simulink model "dpgonio"  (R2019a)
settings: Solver=FixedStepAuto  StartTime=0.0  StopTime=25  RelTol=1e-3  EnableMultiTasking=on
undefined symbols (not defined in the file): Pull, Ts, up
libraries: speedgoatlib_IO183 x5, slrtlib x3, simulink x2
settings Model: Creator=vnalam  LastModifiedBy=vnalam
settings SolverCC: ConcurrentTasks=on  AutoInsertRateTranBlk=on
settings DataIOCC: SaveFormat=StructureWithTime
settings OptimizationCC: BlockReduction=off  OptimizeBlockIOStorage=off  BufferReuse=off  GlobalBufferReuse=off  ExpressionFolding=off  LocalBlockOutputs=off  OptimizeDataStoreBuffers=off  BusAssignmentInplaceUpdate=off
settings HardwareCC: ProdBitPerPointer=32  ProdBitPerSizeT=32  ProdBitPerPtrDiffT=32  ProdLargestAtomicFloat=None  ProdWordSize=32  ProdLongLongMode=on  ProdHWDeviceType=Generic->32-bit x86 compatible
settings RTWCC: SystemTargetFile=slrt.tlc  TemplateMakefile=slrt_default_tmf  Description=Simulink Real-Time  CodeExecutionProfiling=on  RTWCompilerOptimization=on
settings SimulinkRealTimeCC: SupportVariableSizeSignals=on  PreserveStateflowLocalDataDimensions=off  RL32LogTETModifier=off  xPCisDownloadable=off  xPCConcurrentTasks=on

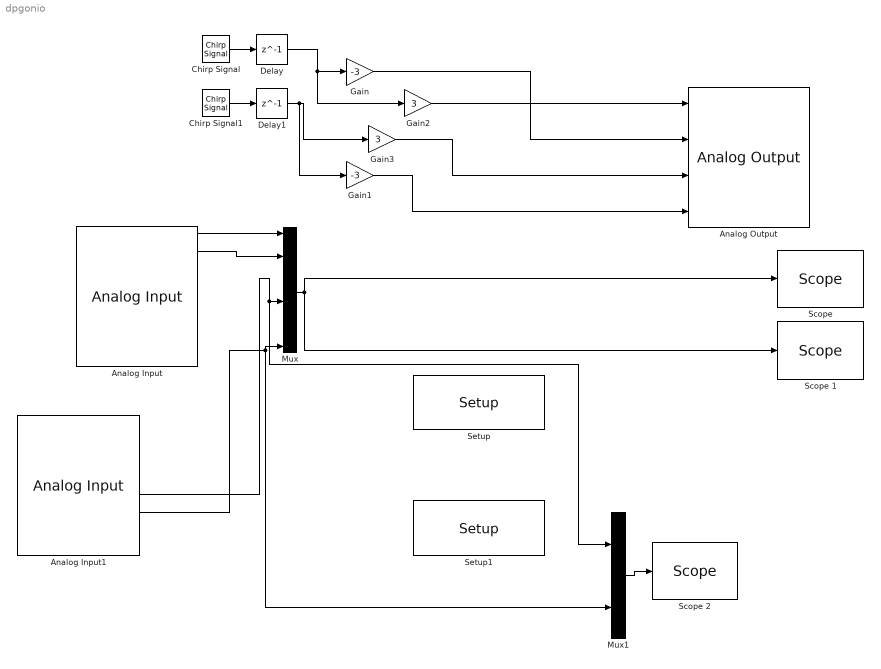
== system dpgonio ==
  Analog Input : speedgoatlib_IO183/Analog Input  Priority=0  parModuleId=1  parSampTime=Ts  parPciSlot=-1  parAdChannelLow=1  parAdChannelHigh=8
      settings: SourceProductName=Simulink Real-Time: Speedgoat Library
  Analog Input1 : speedgoatlib_IO183/Analog Input  Priority=0  parModuleId=2  parSampTime=Ts  parPciSlot=-1  parAdChannelLow=1  parAdChannelHigh=8
      settings: SourceProductName=Simulink Real-Time: Speedgoat Library
  Analog Output : speedgoatlib_IO183/Analog Output  parModuleId=1  parSampTime=-1  parDaSimult=on  parPciSlot=-1  parDaChannels=[1 2 3 4]  parDaInit=[0 0 0 0]  parDaReset=[0 0 0 0]
      settings: SourceProductName=Simulink Real-Time: Speedgoat Library
  Chirp Signal : simulink/Sources/Chirp Signal  f1=0.6  T=25  f2=0.8
  Chirp Signal1 : simulink/Sources/Chirp Signal  f1=0.6  T=25  f2=0.8
  Delay : Delay  DelayLength=1  InitialCondition=0  SampleTime=Ts
  Delay1 : Delay  DelayLength=1  InitialCondition=0  SampleTime=Ts
  Gain : Gain  Gain=-3
  Gain1 : Gain  Gain=-3
  Gain2 : Gain  Gain=3
  Gain3 : Gain  Gain=3
  Mux : Mux  Inputs=6
  Mux1 : Mux  Inputs=2
  "Scope " : slrtlib/Displays and Logging/Scope   scopeno=1  scopetype=Target  autostart=on  viewmode=Graphical sliding  formatstr='%15.6f'  grid=on  ylimits=[0,0]  nosamples=80000  noprepostsamples=0  interleave=1  triggermode=FreeRun  triggersignal=1  trigsignalfromport=off  triggerlevel=0.0  triggerslope=Either  triggerscope=1  triggersample=0  filename=data.dat  mode=Lazy  writesize=512  autorestart=off  dynamicfilemode=off  maxwritefilesize=512*1024^2
  Scope 1 : slrtlib/Displays and Logging/Scope   scopeno=2  scopetype=File  autostart=on  viewmode=Graphical redraw  formatstr='%15.6f'  grid=on  ylimits=[0,0]  nosamples=60000  noprepostsamples=0  interleave=1  triggermode=FreeRun  triggersignal=1  trigsignalfromport=off  triggerlevel=0.0  triggerslope=Either  triggerscope=1  triggersample=0  filename=DPfoot.dat  mode=Commit  writesize=512  autorestart=off  dynamicfilemode=off  maxwritefilesize=512*1024^2
  Scope 2 : slrtlib/Displays and Logging/Scope   scopeno=3  scopetype=Target  autostart=on  viewmode=Graphical sliding  formatstr='%15.6f'  grid=on  ylimits=[0,0]  nosamples=80000  noprepostsamples=0  interleave=1  triggermode=FreeRun  triggersignal=1  trigsignalfromport=off  triggerlevel=0.0  triggerslope=Either  triggerscope=1  triggersample=0  filename=data.dat  mode=Lazy  writesize=512  autorestart=off  dynamicfilemode=off  maxwritefilesize=512*1024^2
  Setup : speedgoatlib_IO183/Setup  parModuleId=1  parPciSlot=-1  parDaSimult=on  parAdCoupling=Single Ended  parAdRange=+-10V  parAdChannelLow=1  parAdChannelHigh=8  parDaChannels=[1:4]  parDaRange=0..5V  parDaInit=[0]  parDaReset=[0]  parDoChannels=[1:8]  parDoInit=[0]  parDoReset=[1]  parDiChannels=[9:16]  parIOPullReferenceFront=Pull-up (3.3V)  parIOPullReferenceRear=Pull-up (3.3V)
      settings: SourceProductName=Simulink Real-Time: Speedgoat Library
  Setup1 : speedgoatlib_IO183/Setup  parModuleId=2  parPciSlot=-1  parDaSimult=on  parAdCoupling=Single Ended  parAdRange=+-10V  parAdChannelLow=1  parAdChannelHigh=8  parDaChannels=[1:4]  parDaRange=0..5V  parDaInit=[0]  parDaReset=[0]  parDoChannels=[1:8]  parDoInit=[0]  parDoReset=[1]  parDiChannels=[9:16]  parIOPullReferenceFront=Pull-up (3.3V)  parIOPullReferenceRear=Pull-up (3.3V)
      settings: SourceProductName=Simulink Real-Time: Speedgoat Library
  wires:
  Mux/1 -> "Scope "/1, Scope 1/1
  Analog Input/2 -> Mux/2
  Analog Input/1 -> Mux/1
  Chirp Signal/1 -> Delay/1
  Chirp Signal1/1 -> Delay1/1
  Delay/1 -> Gain2/1, Gain/1
  Gain/1 -> Analog Output/2
  Delay1/1 -> Gain1/1, Gain3/1
  Gain1/1 -> Analog Output/4
  Gain2/1 -> Analog Output/1
  Gain3/1 -> Analog Output/3
  Analog Input1/5 -> Mux/4, Mux1/1
  Analog Input1/6 -> Mux/6, Mux1/2
  Mux1/1 -> Scope 2/1
